simulink model "pid_test1"  (R2019b)
settings: Solver=FixedStepAuto  StartTime=0.0  StopTime=20  FixedStep=0.01  RelTol=1e-3
settings Model: Creator=subhgang  LastModifiedBy=subhgang

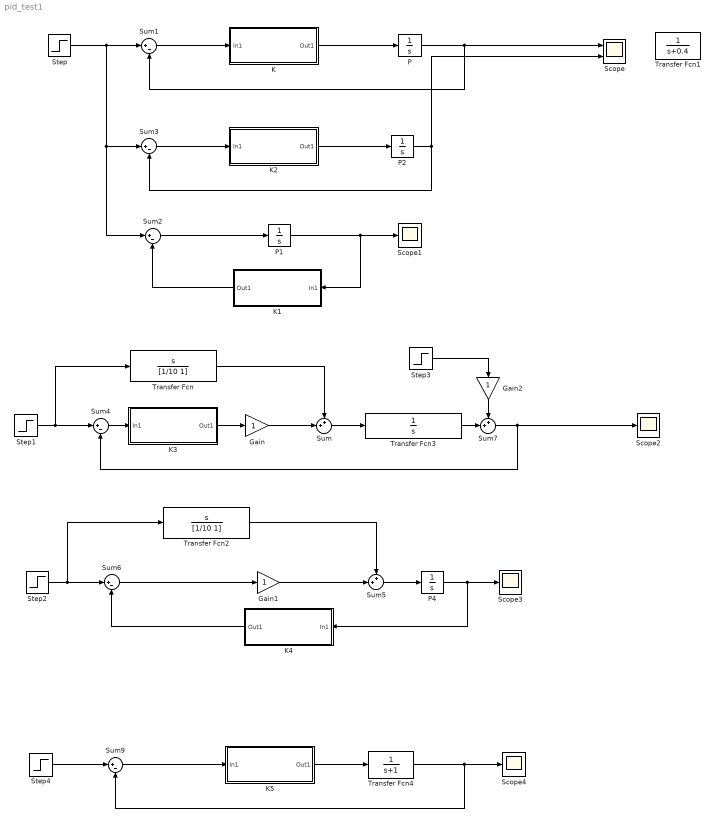
== system pid_test1 ==
  Gain : Gain
  Gain1 : Gain
  Gain2 : Gain
  K : Subsystem
  K1 : Subsystem
  K2 : Subsystem
  K3 : Subsystem
  K4 : Subsystem
  K5 : Subsystem
  P{,1..2,4} (4 alike) : Integrator
  Scope : Scope  NumInputPorts=2
  Scope{1..4} (4 alike) : Scope
  Step{,1..2,4} (4 alike) : Step  SampleTime=0
  Step3 : Step  Time=5  SampleTime=0
  Sum : Sum  Inputs=++|
  Sum{1..4,6,9} (6 alike) : Sum  Inputs=|+-
  Sum5 : Sum  Inputs=++|
  Sum7 : Sum  Inputs=++|
  Transfer Fcn : TransferFcn  Numerator=[1 0]  Denominator=[1/10 1]
  Transfer Fcn1 : TransferFcn  Denominator=[1 0.4]
  Transfer Fcn2 : TransferFcn  Numerator=[1 0]  Denominator=[1/10 1]
  Transfer Fcn3 : TransferFcn  Denominator=[1 0]
  Transfer Fcn4 : TransferFcn  Denominator=[1 1]
  wires:
  Step/1 -> Sum3/1, Sum2/1, Sum1/1
  P/1 -> Scope/1, Sum1/2
  Sum1/1 -> K/1(In1)
  K/1(Out1) -> P/1
  Sum2/1 -> P1/1
  K1/1(Out1) -> Sum2/2
  P1/1 -> Scope1/1, K1/1(In1)
  K2/1(Out1) -> P2/1
  Sum3/1 -> K2/1(In1)
  P2/1 -> Scope/2, Sum3/2
  Step1/1 -> Sum4/1, Transfer Fcn/1
  K3/1(Out1) -> Gain/1
  Transfer Fcn/1 -> Sum/1
  Sum4/1 -> K3/1(In1)
  Gain/1 -> Sum/2
  Gain1/1 -> Sum5/2
  Sum6/1 -> Gain1/1
  Transfer Fcn2/1 -> Sum5/1
  Step2/1 -> Sum6/1, Transfer Fcn2/1
  Sum5/1 -> P4/1
  P4/1 -> K4/1(In1), Scope3/1
  K4/1(Out1) -> Sum6/2
  Sum/1 -> Transfer Fcn3/1
  Sum7/1 -> Sum4/2, Scope2/1
  Step3/1 -> Gain2/1
  Gain2/1 -> Sum7/1
  Transfer Fcn3/1 -> Sum7/2
  K5/1(Out1) -> Transfer Fcn4/1
  Sum9/1 -> K5/1(In1)
  Step4/1 -> Sum9/1
  Transfer Fcn4/1 -> Scope4/1, Sum9/2

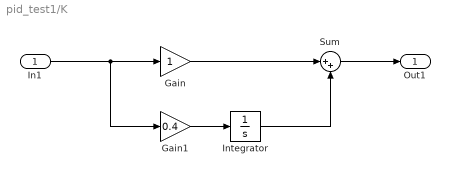
== system pid_test1/K ==
  In1 : Inport
  Gain : Gain
  Gain1 : Gain  Gain=0.4
  Integrator : Integrator
  Sum : Sum  Inputs=|++
  Out1 : Outport
  wires:
  In1/1 -> Gain1/1, Gain/1
  Gain1/1 -> Integrator/1
  Gain/1 -> Sum/1
  Integrator/1 -> Sum/2
  Sum/1 -> Out1/1

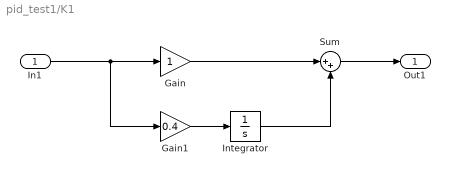
== system pid_test1/K1 ==
  In1 : Inport
  Gain : Gain
  Gain1 : Gain  Gain=0.4
  Integrator : Integrator
  Sum : Sum  Inputs=|++
  Out1 : Outport
  wires:
  Sum/1 -> Out1/1
  Integrator/1 -> Sum/2
  Gain/1 -> Sum/1
  Gain1/1 -> Integrator/1
  In1/1 -> Gain/1, Gain1/1

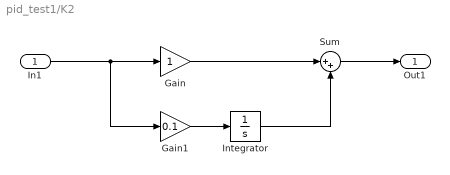
== system pid_test1/K2 ==
  In1 : Inport
  Gain : Gain
  Gain1 : Gain  Gain=0.1
  Integrator : Integrator
  Sum : Sum  Inputs=|++
  Out1 : Outport
  wires:
  Sum/1 -> Out1/1
  Integrator/1 -> Sum/2
  Gain/1 -> Sum/1
  Gain1/1 -> Integrator/1
  In1/1 -> Gain/1, Gain1/1

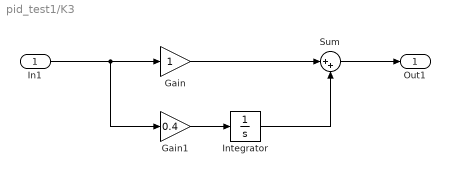
== system pid_test1/K3 ==
  In1 : Inport
  Gain : Gain
  Gain1 : Gain  Gain=0.4
  Integrator : Integrator
  Sum : Sum  Inputs=|++
  Out1 : Outport
  wires:
  In1/1 -> Gain1/1, Gain/1
  Gain1/1 -> Integrator/1
  Gain/1 -> Sum/1
  Integrator/1 -> Sum/2
  Sum/1 -> Out1/1

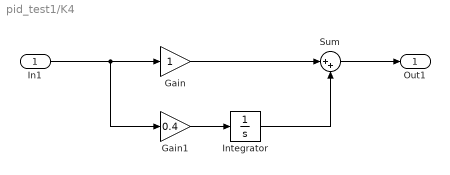
== system pid_test1/K4 ==
  In1 : Inport
  Gain : Gain
  Gain1 : Gain  Gain=0.4
  Integrator : Integrator
  Sum : Sum  Inputs=|++
  Out1 : Outport
  wires:
  In1/1 -> Gain1/1, Gain/1
  Gain1/1 -> Integrator/1
  Gain/1 -> Sum/1
  Integrator/1 -> Sum/2
  Sum/1 -> Out1/1

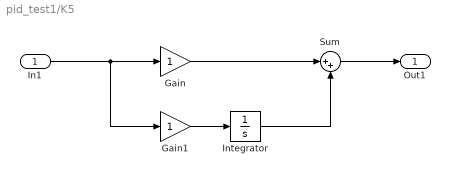
== system pid_test1/K5 ==
  In1 : Inport
  Gain : Gain
  Gain1 : Gain
  Integrator : Integrator
  Sum : Sum  Inputs=|++
  Out1 : Outport
  wires:
  In1/1 -> Gain1/1, Gain/1
  Gain1/1 -> Integrator/1
  Gain/1 -> Sum/1
  Integrator/1 -> Sum/2
  Sum/1 -> Out1/1
